simulink model "teste"  (R2019b)
settings: Solver=VariableStepAuto  StartTime=0.0  StopTime=10  RelTol=1e-3
undefined symbols (not defined in the file): xi
settings Model: Creator=lucas  LastModifiedBy=lucas

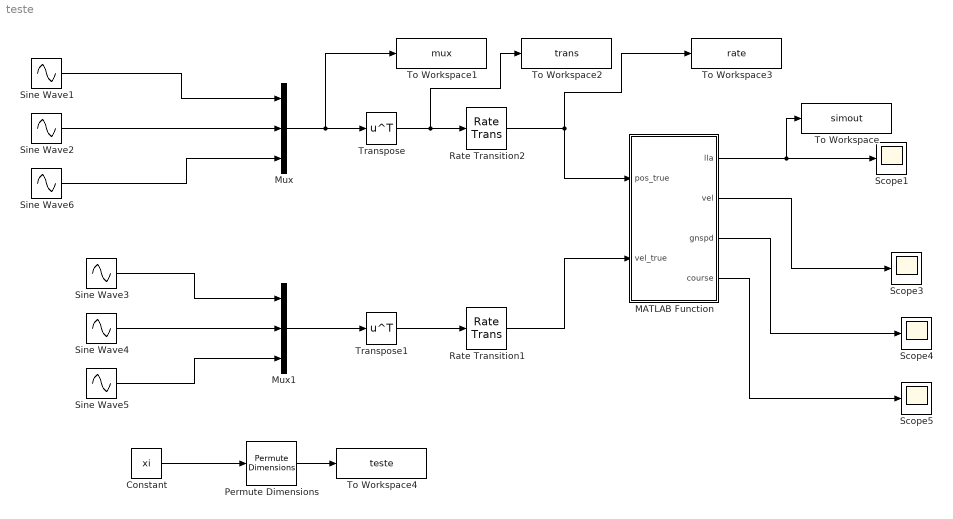
== system teste ==
  Constant : Constant  Value=xi
  MATLAB Function : MATLAB Function  TreatAsAtomicUnit=on
  Mux : Mux  Inputs=3
  Mux1 : Mux  Inputs=3
  Permute Dimensions : PermuteDimensions  Order=[3 2 1]
  Rate Transition1 : RateTransition
  Rate Transition2 : RateTransition
  Scope{1,3..5} (4 alike) : Scope
  Sine Wave{1..6} (6 alike) : Sin  SampleTime=0
  To Workspace : ToWorkspace  VariableName=simout  SaveFormat=Timeseries  SampleTime=-1
  To Workspace1 : ToWorkspace  VariableName=mux  SaveFormat=Timeseries  SampleTime=-1
  To Workspace2 : ToWorkspace  VariableName=trans  SaveFormat=Timeseries  SampleTime=-1
  To Workspace3 : ToWorkspace  VariableName=rate  SaveFormat=Timeseries  SampleTime=-1
  To Workspace4 : ToWorkspace  VariableName=teste  SaveFormat=Timeseries  SampleTime=-1
  Transpose : Math  Operator=transpose  SignedPower=off  SaturateOnIntegerOverflow=on
  Transpose1 : Math  Operator=transpose  SignedPower=off  SaturateOnIntegerOverflow=on
  wires:
  Sine Wave3/1 -> Mux1/1
  Sine Wave4/1 -> Mux1/2
  Sine Wave5/1 -> Mux1/3
  Mux/1 -> To Workspace1/1, Transpose/1
  Mux1/1 -> Transpose1/1
  Transpose/1 -> To Workspace2/1, Rate Transition2/1
  Transpose1/1 -> Rate Transition1/1
  Rate Transition2/1 -> MATLAB Function/1(pos_true), To Workspace3/1
  Rate Transition1/1 -> MATLAB Function/2(vel_true)
  MATLAB Function/2(vel) -> Scope3/1
  MATLAB Function/3(gnspd) -> Scope4/1
  MATLAB Function/4(course) -> Scope5/1
  MATLAB Function/1(lla) -> To Workspace/1, Scope1/1
  Sine Wave1/1 -> Mux/1
  Sine Wave2/1 -> Mux/2
  Sine Wave6/1 -> Mux/3
  Constant/1 -> Permute Dimensions/1
  Permute Dimensions/1 -> To Workspace4/1

== matlab function teste/MATLAB Function ==
  data: pos_true input; lla output; vel_true input; vel output; gnspd output; course output
function [lla, vel, gnspd, course]  = fcn(pos_true, vel_true)

gps = gpsSensor;
gps.VerticalPositionAccuracy = 1.5;


[lla, vel, gnspd, course]  = gps(pos_true, vel_true);

end
